simulink model "BoostRollSIL"  (R2026a)
settings: Solver=FixedStepDiscrete  StopTime=8  FixedStep=0.0025
PreLoadFcn:
  | boost_roll_slx_setup
InitFcn:
  | clear boost_roll_plant_pack boost_roll_ctrl_pack; boost_roll_slx_setup
undefined symbols (not defined in the file or in its folder): boost_p
settings Model: Creator=vhalii  LastModifiedBy=vhalii

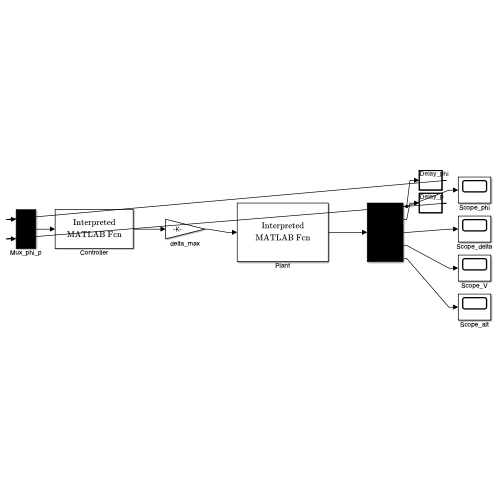
[thumbnail: Simulink's stored preview of the top-level diagram]
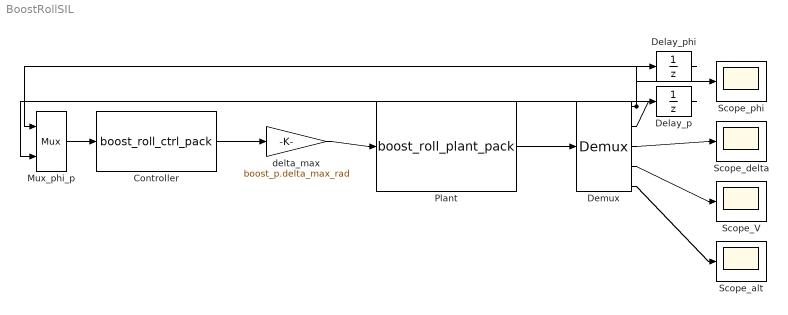
== system BoostRollSIL ==
  Controller : MATLABFcn  MATLABFcn=boost_roll_ctrl_pack
  Delay_p : UnitDelay  SampleTime=0.0025
  Delay_phi : UnitDelay  SampleTime=0.0025
  Demux : Demux  Outputs=5
  Mux_phi_p : Mux  Inputs=2
  Plant : MATLABFcn  MATLABFcn=boost_roll_plant_pack  OutputDimensions=5
  Scope_V : Scope
  Scope_alt : Scope
  Scope_delta : Scope
  Scope_phi : Scope
  delta_max : Gain  Gain=boost_p.delta_max_rad
  wires:
  Mux_phi_p/1 -> Controller/1
  Controller/1 -> delta_max/1
  delta_max/1 -> Plant/1
  Plant/1 -> Demux/1
  Demux/1 -> Scope_phi/1, Delay_phi/1
  Demux/3 -> Scope_delta/1
  Demux/4 -> Scope_V/1
  Demux/5 -> Scope_alt/1
  Demux/2 -> Delay_p/1
  Delay_phi/1 -> Mux_phi_p/1
  Delay_p/1 -> Mux_phi_p/2
